simulink model "Controller_sim2020"  (R2020b)
settings: Solver=VariableStepAuto  StartTime=0.0  StopTime=30  RelTol=1e-3
values from neighbouring files (symbols this model uses):
  F_mimo = -place(sysd.A,sysd.B,Desired_poles)    [SS_MIMO.m]    (also in workspace.mat = [-1.46285714286 0 0 0 0 -3.44816326531 0 0 0 0 -3.0563265306)
  L_mimo = -place(sysd.A',sysd.C',Desired_poles_obs)'    [SS_MIMO.m]    (also in workspace.mat = [-2 0 0 0 0 0 0 0 0 -1.85714285714 0 0 ... (64 elements, 8x8)
  M = [3.75 0 0 0 2.57142857143 0 0 0 0 0.0633116883117 0 0 ... (64 elements, 8x8)]    [workspace.mat]
  N = [3.65714285714 0 0 0 0 3.05632653061 0 0 0 0 2.50775510204 0 ... (32 elements, 4x8)]    [workspace.mat]
  sys_mimo = ss(A,B,C,0)    [SS_MIMO.m]
libraries: simulink_extras x6, simulink x1
settings Model: Creator=krist  LastModifiedBy=mozzr

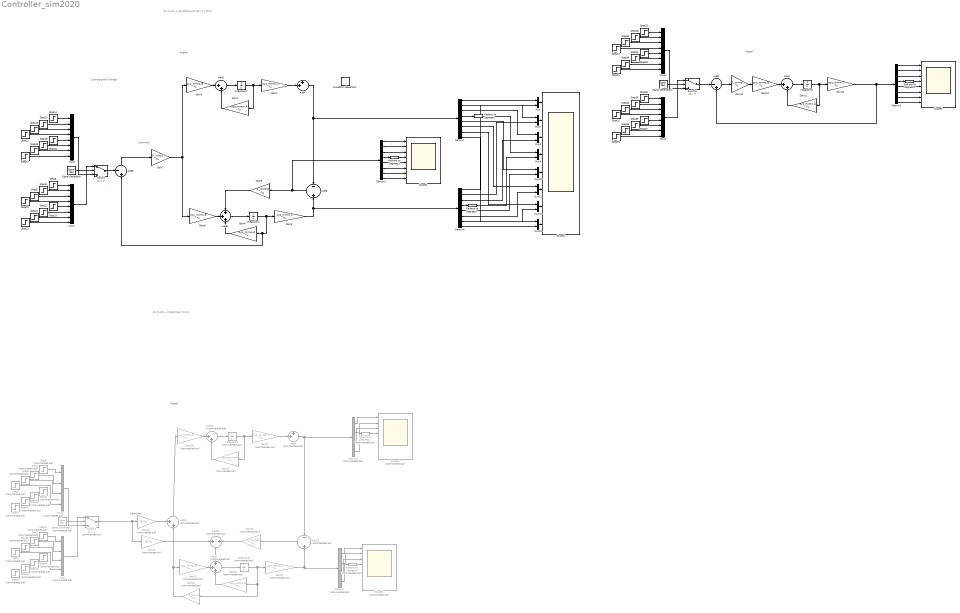
== system Controller_sim2020 ==
  note: Ragnar
  note: Controller
  note: Controlsignal
      | to Rangar
  note: dX = A*X + [0;1/M]*pinv(J')*ta
      | Y = J'*C*X
  note: dX = A*X + [0;1/M]*Fa
      | Y = C*X
  note: Ragnar
  note: Ragnar
  note: Controller
  Add1 : Sum  Inputs=|++
  Add10 : Sum  Commented=on  Inputs=|++
  Add11 : Sum  Commented=on  Inputs=+++
  Add12 : Sum  Commented=on
  Add13 : Sum  Commented=on  Inputs=-+
  Add14 : Sum  Commented=on  Inputs=++|
  Add2 : Sum  Inputs=|-+
  Add3 : Sum  Commented=on  Inputs=++|
  Add4 : Sum  Inputs=++|
  Add5 : Sum  Inputs=|++
  Add6 : Sum  Inputs=+++
  Add8 : Sum  Inputs=-+
  Add9 : Sum  Inputs=-+|
  Demux1 : Demux  Commented=on
  Demux{2..3,6..7} (4 alike) : Demux  Outputs=8
  Demux5 : Demux  Commented=on
  Gain1 : Gain  Gain=sys_mimo.A  Multiplication=Matrix(K*u)
  Gain11 : Gain  Gain=sys_mimo.A  Multiplication=Matrix(K*u)
  Gain12 : Gain  Gain=sys_mimo.C  Multiplication=Matrix(K*u)
  Gain13 : Gain  Gain=sys_mimo.B  Multiplication=Matrix(K*u)
  Gain14 : Gain  Gain=F_mimo  Multiplication=Matrix(K*u)
  Gain15 : Gain  Commented=on  Gain=sys_mimo.A  Multiplication=Matrix(K*u)
  Gain16 : Gain  Commented=on  Gain=M  Multiplication=Matrix(K*u)
  Gain17 : Gain  Commented=on  Gain=sys_mimo.C  Multiplication=Matrix(K*u)
  Gain18 : Gain  Commented=on  Gain=sys_mimo.B  Multiplication=Matrix(K*u)
  Gain19 : Gain  Commented=on  Gain=sys_mimo.A  Multiplication=Matrix(K*u)
  Gain2 : Gain  Gain=sys_mimo.C  Multiplication=Matrix(K*u)
  Gain20 : Gain  Commented=on  Gain=sys_mimo.C  Multiplication=Matrix(K*u)
  Gain21 : Gain  Commented=on  Gain=sys_mimo.B  Multiplication=Matrix(K*u)
  Gain22 : Gain  Commented=on  Gain=F_mimo  Multiplication=Matrix(K*u)
  Gain23 : Gain  Commented=on  Gain=L_mimo  Multiplication=Matrix(K*u)
  Gain24 : Gain  Commented=on  Gain=N  Multiplication=Matrix(K*u)
  Gain3 : Gain  Gain=sys_mimo.B  Multiplication=Matrix(K*u)
  Gain4 : Gain  Gain=sys_mimo.A  Multiplication=Matrix(K*u)
  Gain5 : Gain  Gain=sys_mimo.C  Multiplication=Matrix(K*u)
  Gain6 : Gain  Gain=sys_mimo.B  Multiplication=Matrix(K*u)
  Gain7 : Gain  Gain=F_mimo  Multiplication=Matrix(K*u)
  Gain8 : Gain  Gain=L_mimo  Multiplication=Matrix(K*u)
  Integrator1 : Integrator  InitialCondition=[0 0.5 -0.4 deg2rad(90) 0 0 0 0]
  Integrator2 : Integrator  InitialCondition=[0 0.5 -0.4 deg2rad(90) 0 0 0 0]
  Integrator3 : Integrator  Commented=on  InitialCondition=[0 0.5 -0.4 deg2rad(90) 0 0 0 0]
  Integrator4 : Integrator  InitialCondition=[0 0.55 -0.35 deg2rad(93) 0 0 0 0]
  Integrator5 : Integrator  Commented=on  InitialCondition=[0 0.5 -0.4 deg2rad(90) 0 0 0 0]
  Mux{,7..13} (8 alike) : Mux  Inputs=2
  Mux1 : Mux  Commented=on
  Mux{2..3,5..6} (4 alike) : Mux  Inputs=8
  Mux4 : Mux  Commented=on
  Radians to Degrees1 : simulink_extras/Transformations/Radians to Degrees  Commented=on
  Radians to Degrees{2..3,6..7} (4 alike) : simulink_extras/Transformations/Radians to Degrees
  Radians to Degrees5 : simulink_extras/Transformations/Radians to Degrees  Commented=on
  Scope1 : Scope  Commented=on  NumInputPorts=8
  Scope2 : Scope  NumInputPorts=8
  Scope3 : Scope  NumInputPorts=8
  Scope4 : Scope  NumInputPorts=8
  Scope5 : Scope  Commented=on  NumInputPorts=8
  Signal Generator : SignalGenerator  WaveForm=square  Frequency=0.4  Units=rad/sec
  Signal Generator1 : SignalGenerator  Commented=on  WaveForm=square  Frequency=0.4  Units=rad/sec
  Signal Generator2 : SignalGenerator  WaveForm=square  Frequency=0.4  Units=rad/sec
  Step1 : Step  Commented=on  Time=0  Before=deg2rad(85)  After=deg2rad(85)  SampleTime=1
  Step10 : Step  Time=0  Before=deg2rad(85)  After=deg2rad(85)  SampleTime=1
  Step11 : Step  Time=0  Before=0.51  After=0.51  SampleTime=1
  Step12 : Step  Time=0  Before=deg2rad(90)  After=deg2rad(90)  SampleTime=1
  Step13 : Step  Time=0  Before=0.5  After=0.5  SampleTime=1
  Step{14,17..24,29,31..38} (18 alike) : Step  Time=0  After=0  SampleTime=1
  Step15 : Step  Time=0  Before=-0.4  After=-0.4  SampleTime=1
  Step{5,7,16,41..46} (9 alike) : Step  Commented=on  Time=0  After=0  SampleTime=1
  Step2 : Step  Commented=on  Time=0  Before=0.51  After=0.51  SampleTime=1
  Step25 : Step  Time=0  Before=deg2rad(85)  After=deg2rad(85)  SampleTime=1
  Step26 : Step  Time=0  Before=0.51  After=0.51  SampleTime=1
  Step27 : Step  Time=0  Before=deg2rad(90)  After=deg2rad(90)  SampleTime=1
  Step28 : Step  Time=0  Before=0.5  After=0.5  SampleTime=1
  Step3 : Step  Commented=on  Time=0  Before=deg2rad(90)  After=deg2rad(90)  SampleTime=1
  Step30 : Step  Time=0  Before=-0.4  After=-0.4  SampleTime=1
  Step39 : Step  Time=0  Before=0.01  After=0.01  SampleTime=1
  Step4 : Step  Commented=on  Time=0  Before=0.5  After=0.5  SampleTime=1
  Step40 : Step  Time=0  Before=-0.41  After=-0.41  SampleTime=1
  Step47 : Step  Commented=on  Time=0  Before=0.01  After=0.01  SampleTime=1
  Step48 : Step  Commented=on  Time=0  Before=-0.41  After=-0.41  SampleTime=1
  Step6 : Step  Commented=on  Time=0  Before=-0.4  After=-0.4  SampleTime=1
  Step8 : Step  Time=0  Before=0.01  After=0.01  SampleTime=1
  Step9 : Step  Time=0  Before=-0.41  After=-0.41  SampleTime=1
  Switch : Switch  Criteria=u2 > Threshold
  Switch1 : Switch  Commented=on  Criteria=u2 > Threshold
  Switch2 : Switch  Criteria=u2 > Threshold
  Waveform Generator : simulink/Sources/Waveform Generator  OutMin=[]  OutMax=[]  OutDataTypeStr=double  SelectedSignal=8  Signals=gaussian(0,0.1,123)#gaussian(0,0.1,123)#gaussian(0,0.1,123)#gaussian(0,0.1,123)#gaussian(0,0.1,123)#gaussian(0,0.1,123)#gaussian(0,0.1,123)#gaussian(0,0.1,123)  BlockNames=MultiportSwitch_7063c7644348442#MultiportSwitch_7a0bf61efa1946a#MultiportSwitch_1a360fe1297541d#MultiportSwitch_36fbd782c0784f7#MultiportSwitch_8af81a1dd9874d2#MultiportSwitch_0411fe225a18433#MultiportSwitch_fcf9c4fc37514ba#MultiportSwitch_69608ae098394aa  SampleTime=0.1
  wires:
  Add8/1 -> Demux3/1, Gain8/1
  Gain1/1 -> Add5/2
  Integrator1/1 -> Gain1/1, Gain2/1
  Add5/1 -> Integrator1/1
  Gain3/1 -> Add5/1
  Switch/1 -> Add9/1
  Add6/1 -> Integrator4/1
  Gain4/1 -> Add6/3
  Gain8/1 -> Add6/1
  Gain6/1 -> Add6/2
  Signal Generator/1 -> Switch/2
  Step10/1 -> Mux2/4
  Step9/1 -> Mux2/3
  Step8/1 -> Mux2/1
  Step11/1 -> Mux2/2
  Step12/1 -> Mux3/4
  Step15/1 -> Mux3/3
  Step14/1 -> Mux3/1
  Step13/1 -> Mux3/2
  Mux2/1 -> Switch/1
  Mux3/1 -> Switch/3
  Gain13/1 -> Add1/1
  Gain11/1 -> Add1/2
  Add1/1 -> Integrator2/1
  Integrator2/1 -> Gain11/1, Gain12/1
  Gain12/1 -> Add2/2, Demux2/1
  Demux2/4 -> Radians to Degrees2/1
  Demux2/3 -> Scope3/3
  Demux2/2 -> Scope3/2
  Demux2/1 -> Scope3/1
  Demux2/5 -> Scope3/5
  Demux2/6 -> Scope3/6
  Demux2/8 -> Scope3/8
  Demux2/7 -> Scope3/7
  Radians to Degrees2/1 -> Scope3/4
  Step18/1 -> Mux3/6
  Step17/1 -> Mux3/8
  Step20/1 -> Mux3/7
  Step19/1 -> Mux3/5
  Step23/1 -> Mux2/5
  Step22/1 -> Mux2/6
  Step24/1 -> Mux2/7
  Step21/1 -> Mux2/8
  Integrator4/1 -> Add9/2, Gain4/1, Gain5/1
  Gain2/1 -> Add4/2
  Add2/1 -> Gain14/1
  Gain14/1 -> Gain13/1
  Step28/1 -> Mux6/2
  Step26/1 -> Mux5/2
  Signal Generator2/1 -> Switch2/2
  Step27/1 -> Mux6/4
  Step34/1 -> Mux6/7
  Mux5/1 -> Switch2/1
  Step39/1 -> Mux5/1
  Step38/1 -> Mux5/7
  Step29/1 -> Mux6/1
  Step35/1 -> Mux5/8
  Step37/1 -> Mux5/5
  Step40/1 -> Mux5/3
  Step25/1 -> Mux5/4
  Step33/1 -> Mux6/5
  Step36/1 -> Mux5/6
  Switch2/1 -> Add2/1
  Step31/1 -> Mux6/8
  Step30/1 -> Mux6/3
  Step32/1 -> Mux6/6
  Mux6/1 -> Switch2/3
  Gain17/1 -> Add3/2
  Add3/1 -> Demux5/1, Add13/1
  Demux1/1 -> Scope1/1
  Radians to Degrees1/1 -> Scope5/4
  Add11/1 -> Integrator5/1
  Demux1/2 -> Scope1/2
  Signal Generator1/1 -> Switch1/2
  Step2/1 -> Mux1/2
  Step3/1 -> Mux4/4
  Gain18/1 -> Add10/1
  Mux4/1 -> Switch1/3
  Gain21/1 -> Add11/2
  Add12/1 -> Add11/1
  Gain24/1 -> Add14/1
  Step6/1 -> Mux4/3
  Gain19/1 -> Add11/3
  Add10/1 -> Integrator3/1
  Step1/1 -> Mux1/4
  Step48/1 -> Mux1/3
  Mux1/1 -> Switch1/1
  Gain20/1 -> Demux1/1, Add13/2
  Gain15/1 -> Add10/2
  Add14/1 -> Gain18/1
  Demux5/2 -> Scope5/2
  Integrator5/1 -> Gain19/1, Gain22/1, Gain20/1
  Step4/1 -> Mux4/2
  Switch1/1 -> Gain16/1, Gain24/1
  Step5/1 -> Mux4/1
  Gain16/1 -> Add12/1
  Gain22/1 -> Gain21/1, Add14/2
  Demux5/3 -> Scope5/3
  Add13/1 -> Gain23/1
  Demux1/4 -> Radians to Degrees5/1
  Integrator3/1 -> Gain15/1, Gain17/1
  Demux1/3 -> Scope1/3
  Radians to Degrees5/1 -> Scope1/4
  Demux5/4 -> Radians to Degrees1/1
  Gain23/1 -> Add12/2
  Step47/1 -> Mux1/1
  Demux5/1 -> Scope5/1
  Gain5/1 -> Add8/2, Demux6/1
  Demux7/8 -> Mux13/1
  Demux7/3 -> Mux8/1
  Demux7/2 -> Mux7/1
  Add4/1 -> Add8/1, Demux7/1
  Demux7/1 -> Mux/1
  Demux7/4 -> Radians to Degrees6/1
  Demux6/4 -> Radians to Degrees7/1
  Mux/1 -> Scope4/1
  Mux7/1 -> Scope4/2
  Mux8/1 -> Scope4/3
  Mux9/1 -> Scope4/4
  Mux13/1 -> Scope4/8
  Mux12/1 -> Scope4/7
  Mux10/1 -> Scope4/5
  Mux11/1 -> Scope4/6
  Radians to Degrees6/1 -> Mux9/1
  Demux7/5 -> Mux10/1
  Demux7/6 -> Mux11/1
  Demux7/7 -> Mux12/1
  Demux6/8 -> Mux13/2
  Demux6/7 -> Mux12/2
  Demux6/6 -> Mux11/2
  Demux6/5 -> Mux10/2
  Radians to Degrees7/1 -> Mux9/2
  Demux6/3 -> Mux8/2
  Demux6/2 -> Mux7/2
  Demux6/1 -> Mux/2
  Demux3/6 -> Scope2/6
  Demux3/7 -> Scope2/7
  Demux3/1 -> Scope2/1
  Demux3/2 -> Scope2/2
  Demux3/4 -> Radians to Degrees3/1
  Radians to Degrees3/1 -> Scope2/4
  Demux3/8 -> Scope2/8
  Demux3/3 -> Scope2/3
  Demux3/5 -> Scope2/5
  Add9/1 -> Gain7/1
  Gain7/1 -> Gain6/1, Gain3/1
